simulink model "suspension_control_system"  (R2012b)
settings: Solver=ode3  SolverMode=SingleTasking  StartTime=0.0  StopTime=30  FixedStep=T  RelTol=1e-3
PreLoadFcn:
  | init_parameters;
undefined symbols (not defined in the file): K_lqr, opy_full, Suspension, sys_estimator
libraries: vehicle_dynamics_lib x7
settings Model: Creator=Marcus Sonntag  LastModifiedBy=vikafla
settings SolverCC: ZeroCrossAlgorithm=Adaptive
settings DataIOCC: SignalLoggingSaveFormat=ModelDataLogs  SaveOutput=off  SignalLogging=off  SaveTime=off
settings OptimizationCC: InlineParams=on  UseIntDivNetSlope=on  InlineInvariantSignals=on  EnhancedBackFolding=on  EfficientFloat2IntCast=on  SimCompilerOptimization=On
settings DebuggingCC: ArtificialAlgebraicLoopMsg=none  ParameterTunabilityLossMsg=none  FcnCallInpInsideContextMsg=UseLocalSettings  UniqueDataStoreMsg=error  StrictBusMsg=Warning
settings HardwareCC: ProdHWDeviceType=Generic->Unspecified (assume 32-bit Generic)  TargetIntDivRoundTo=Zero  TargetEndianess=LittleEndian  TargetHWDeviceType=Atmel->AVR
settings SFSimCC: SimParseCustomCode=off
settings RTWCC: SystemTargetFile=cn.tlc  TemplateMakefile=cn_msdll.tmf  PostCodeGenCommand=packNGo(buildInfo, {'packType' 'hierarchical'})  Description=Vector CANoe Real-Time Target DLL (Visual C/C++ Project Makefile)  ProcessScript=cn_make_rtw_hook  RTWCompilerOptimization=On
settings CodeAppCC: GenerateComments=off  MaxIdLength=128  SimulinkBlockComments=off
settings STFCustomTargetCC: CodeReplacementLibrary=ANSI_C  GeneratePreprocessorConditionals=Disable all  MatFileLogging=on  SystemTargetFile=cn.tlc
settings GRTTargetCC: ParMdlRefBuildCompliant=off  CompOptLevelCompliant=off  ConcurrentExecutionCompliant=off  CombineOutputUpdateFcns=off  GRTInterface=on  ExtModeMexFile=noextcomm  RTWCAPISignals=on  RTWCAPIParams=on

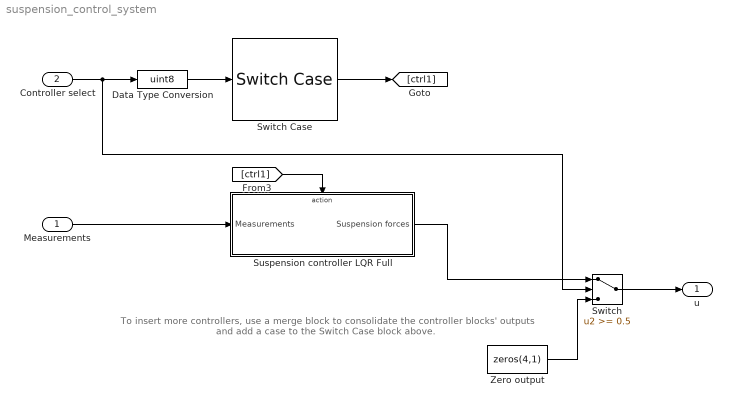
== system suspension_control_system ==
  note: To insert more controllers, use a merge block to consolidate
      | the controller blocks' outputs and add a case to the Switch Case
      | block above.
  Measurements : Inport  OutDataTypeStr=Bus: Bus_Measurements
  Controller select : Inport  Port=2
  Data Type Conversion : DataTypeConversion  OutDataTypeStr=uint8
  Suspension controller LQR Full : Subsystem
  Switch : Switch  Threshold=0.5
  Switch Case : SwitchCase  ShowDefaultCase=off
  Zero output : Constant  Value=zeros(4,1)
  u : Outport
  wires:
  Measurements/1 -> Suspension controller LQR Full/1(Measurements)
  Controller select/1 -> Data Type Conversion/1, Switch/2
  Switch Case/1 -> [ctrl1]
  [ctrl1] -> Suspension controller LQR Full/Action
  Data Type Conversion/1 -> Switch Case/1
  Suspension controller LQR Full/1(Suspension forces) -> Switch/1
  Switch/1 -> u/1
  Zero output/1 -> Switch/3

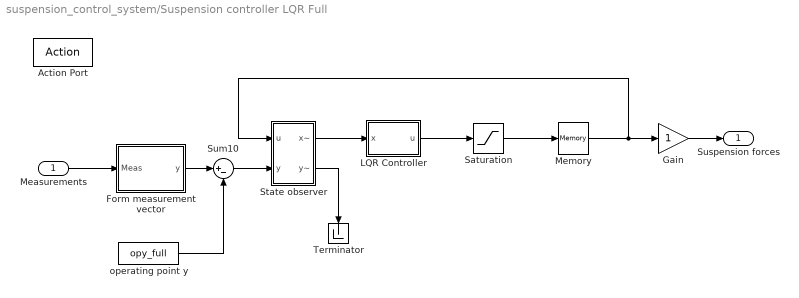
== system suspension_control_system/Suspension controller LQR Full ==
  Measurements : Inport
  Action Port : ActionPort  ActionType=case
  Form measurement vector : Subsystem
  Gain : Gain
  LQR Controller : Subsystem
  Memory : Memory
  Saturation : Saturate  UpperLimit=6e3  LowerLimit=-6e3
  State observer : Subsystem
  Sum10 : Sum  Inputs=|+-
  Terminator : Terminator
  operating point y : Constant  Value=opy_full
  Suspension forces : Outport  OutDataTypeStr=double  PortDimensions=4
  wires:
  LQR Controller/1(u) -> Saturation/1
  State observer/2(y~) -> Terminator/1
  Gain/1 -> Suspension forces/1
  State observer/1(x~) -> LQR Controller/1(x)
  Measurements/1 -> Form measurement vector/1(Meas)
  Form measurement vector/1(y) -> Sum10/1
  operating point y/1 -> Sum10/2
  Sum10/1 -> State observer/2(y)
  Saturation/1 -> Memory/1
  Memory/1 -> Gain/1, State observer/1(u)

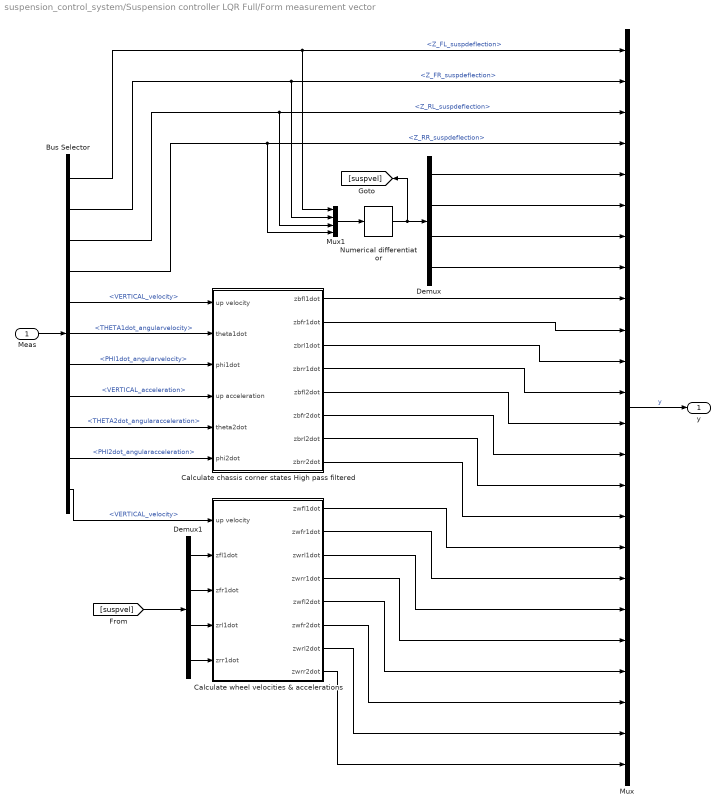
== system suspension_control_system/Suspension controller LQR Full/Form measurement vector ==
  Meas : Inport
  Bus Selector : BusSelector  OutputSignals=Z_FL_suspdeflection,Z_FR_suspdeflection,Z_RL_suspdeflection,Z_RR_suspdeflection,VERTICAL_velocity,THETA1dot_angularvelocity,PHI1dot_angularvelocity,VERTICAL_acceleration,THETA2dot_angularacceleration,PHI2dot_angularacceleration,VERTICAL_velocity
  Calculate chassis corner states High pass filtered : Subsystem
  Calculate wheel velocities & accelerations : Subsystem
  Demux : Demux
  Demux1 : Demux
  Mux : Mux  Inputs=24
  Mux1 : Mux
  Numerical differentiator : vehicle_dynamics_lib/Helper blocks/Numerical differentiator  SystemSampleTime=-1  Ts=0.01
  y : Outport
  wires:
  [suspvel] -> Demux1/1
  Demux1/4 -> Calculate wheel velocities & accelerations/5(zrr1dot)
  Demux1/3 -> Calculate wheel velocities & accelerations/4(zrl1dot)
  Demux1/2 -> Calculate wheel velocities & accelerations/3(zfr1dot)
  Demux1/1 -> Calculate wheel velocities & accelerations/2(zfl1dot)
  Demux/4 -> Mux/8
  Demux/3 -> Mux/7
  Demux/2 -> Mux/6
  Demux/1 -> Mux/5
  Numerical differentiator/1 -> [suspvel], Demux/1
  Mux1/1 -> Numerical differentiator/1
  Calculate wheel velocities & accelerations/8(zwrr2dot) -> Mux/24
  Calculate wheel velocities & accelerations/7(zwrl2dot) -> Mux/23
  Calculate wheel velocities & accelerations/6(zwfr2dot) -> Mux/22
  Calculate wheel velocities & accelerations/5(zwfl2dot) -> Mux/21
  Calculate wheel velocities & accelerations/4(zwrr1dot) -> Mux/20
  Calculate wheel velocities & accelerations/3(zwrl1dot) -> Mux/19
  Calculate wheel velocities & accelerations/2(zwfr1dot) -> Mux/18
  Calculate wheel velocities & accelerations/1(zwfl1dot) -> Mux/17
  Bus Selector/11 -> Calculate wheel velocities & accelerations/1(up velocity)  "<VERTICAL_velocity>"
  Calculate chassis corner states High pass filtered/8(zbrr2dot) -> Mux/16
  Calculate chassis corner states High pass filtered/7(zbrl2dot) -> Mux/15
  Calculate chassis corner states High pass filtered/6(zbfr2dot) -> Mux/14
  Calculate chassis corner states High pass filtered/5(zbfl2dot) -> Mux/13
  Calculate chassis corner states High pass filtered/4(zbrr1dot) -> Mux/12
  Calculate chassis corner states High pass filtered/3(zbrl1dot) -> Mux/11
  Calculate chassis corner states High pass filtered/2(zbfr1dot) -> Mux/10
  Calculate chassis corner states High pass filtered/1(zbfl1dot) -> Mux/9
  Bus Selector/10 -> Calculate chassis corner states High pass filtered/6(phi2dot)  "<PHI2dot_angularacceleration>"
  Bus Selector/7 -> Calculate chassis corner states High pass filtered/3(phi1dot)  "<PHI1dot_angularvelocity>"
  Bus Selector/4 -> Mux1/4, Mux/4  "<Z_RR_suspdeflection>"
  Bus Selector/3 -> Mux1/3, Mux/3  "<Z_RL_suspdeflection>"
  Bus Selector/2 -> Mux1/2, Mux/2  "<Z_FR_suspdeflection>"
  Bus Selector/1 -> Mux1/1, Mux/1  "<Z_FL_suspdeflection>"
  Bus Selector/5 -> Calculate chassis corner states High pass filtered/1(up velocity)  "<VERTICAL_velocity>"
  Bus Selector/6 -> Calculate chassis corner states High pass filtered/2(theta1dot)  "<THETA1dot_angularvelocity>"
  Bus Selector/9 -> Calculate chassis corner states High pass filtered/5(theta2dot)  "<THETA2dot_angularacceleration>"
  Bus Selector/8 -> Calculate chassis corner states High pass filtered/4(up acceleration)  "<VERTICAL_acceleration>"
  Meas/1 -> Bus Selector/1
  Mux/1 -> y/1  "y"

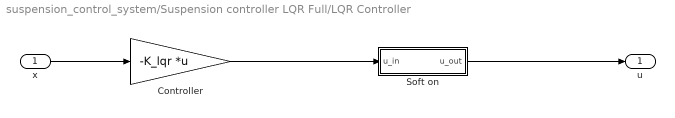
== system suspension_control_system/Suspension controller LQR Full/LQR Controller ==
  x : Inport  PortDimensions=14
  Controller : Gain  Gain=-K_lqr  Multiplication=Matrix(K*u)
  Soft on : Subsystem
  u : Outport
  wires:
  Soft on/1(u_out) -> u/1
  x/1 -> Controller/1
  Controller/1 -> Soft on/1(u_in)

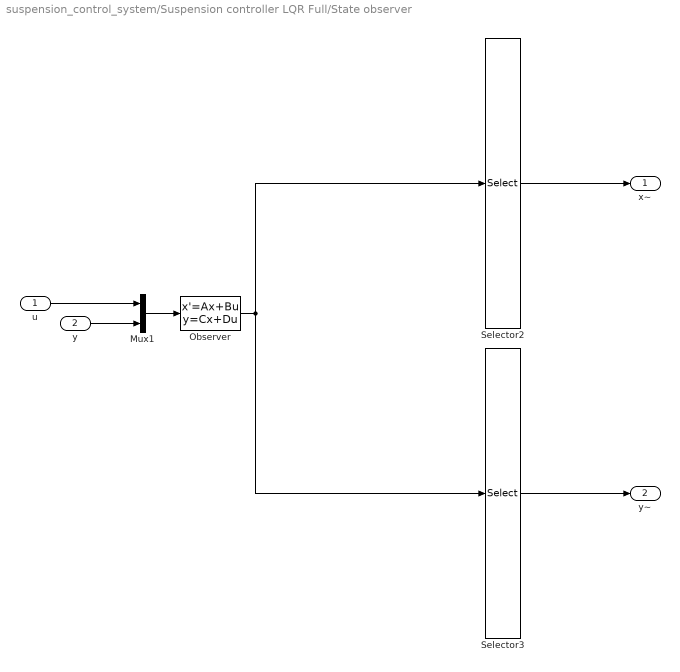
== system suspension_control_system/Suspension controller LQR Full/State observer ==
  u : Inport
  y : Inport  Port=2
  Mux1 : Mux  Inputs=2
  Observer : StateSpace  A=sys_estimator.A  B=sys_estimator.B  C=sys_estimator.C  D=sys_estimator.D  X0=zeros(14,1)
  Selector2 : Selector  InputPortWidth=size(sys_estimator.C,1)  IndexOptions=Index vector (dialog)  Indices=[(size(sys_estimator.C,1)-size(sys_estimator.A,1)+1):(size(sys_estimator.C,1))]  OutputSizes=1
  Selector3 : Selector  InputPortWidth=size(sys_estimator.C,1)  IndexOptions=Index vector (dialog)  Indices=[1:size(sys_estimator.C,1)-size(sys_estimator.A,1)]  OutputSizes=1
  x~ : Outport
  y~ : Outport  Port=2
  wires:
  Selector2/1 -> x~/1
  Selector3/1 -> y~/1
  Observer/1 -> Selector2/1, Selector3/1
  y/1 -> Mux1/2
  u/1 -> Mux1/1
  Mux1/1 -> Observer/1

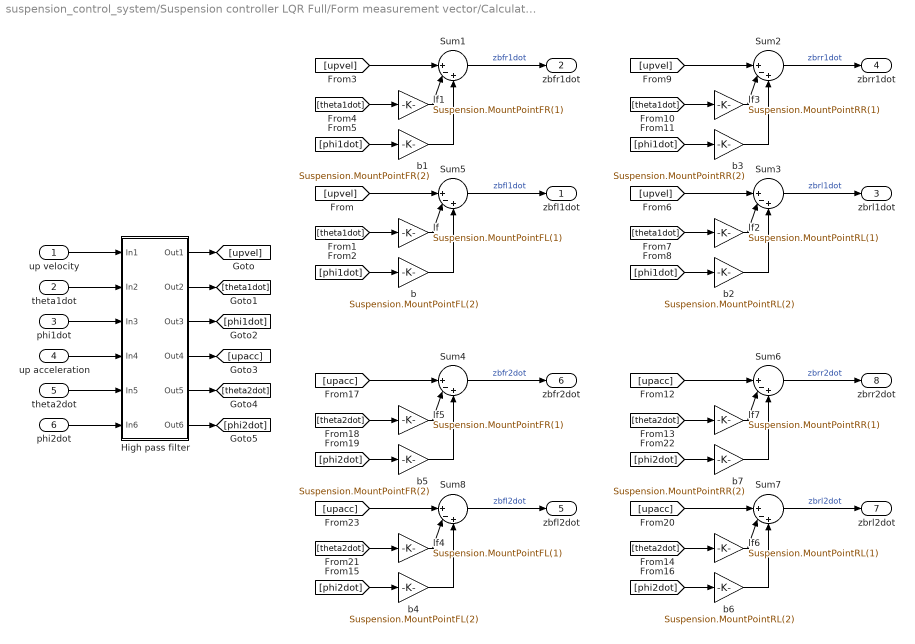
== system suspension_control_system/Suspension controller LQR Full/Form measurement vector/Calculate chassis corner states High pass filtered ==
  up velocity : Inport
  theta1dot : Inport  Port=2
  phi1dot : Inport  Port=3
  up acceleration : Inport  Port=4
  theta2dot : Inport  Port=5
  phi2dot : Inport  Port=6
  High pass filter : Subsystem
  Sum{1..8} (8 alike) : Sum  Inputs=||+-+
  b : Gain  Gain=Suspension.MountPointFL(2)
  b1 : Gain  Gain=Suspension.MountPointFR(2)
  b2 : Gain  Gain=Suspension.MountPointRL(2)
  b3 : Gain  Gain=Suspension.MountPointRR(2)
  b4 : Gain  Gain=Suspension.MountPointFL(2)
  b5 : Gain  Gain=Suspension.MountPointFR(2)
  b6 : Gain  Gain=Suspension.MountPointRL(2)
  b7 : Gain  Gain=Suspension.MountPointRR(2)
  lf : Gain  Gain=Suspension.MountPointFL(1)
  lf1 : Gain  Gain=Suspension.MountPointFR(1)
  lf2 : Gain  Gain=Suspension.MountPointRL(1)
  lf3 : Gain  Gain=Suspension.MountPointRR(1)
  lf4 : Gain  Gain=Suspension.MountPointFL(1)
  lf5 : Gain  Gain=Suspension.MountPointFR(1)
  lf6 : Gain  Gain=Suspension.MountPointRL(1)
  lf7 : Gain  Gain=Suspension.MountPointRR(1)
  zbfl1dot : Outport
  zbfr1dot : Outport  Port=2
  zbrl1dot : Outport  Port=3
  zbrr1dot : Outport  Port=4
  zbfl2dot : Outport  Port=5
  zbfr2dot : Outport  Port=6
  zbrl2dot : Outport  Port=7
  zbrr2dot : Outport  Port=8
  wires:
  [theta2dot] -> lf7/1
  [phi2dot] -> b7/1
  [upacc] -> Sum6/1
  b7/1 -> Sum6/3
  Sum6/1 -> zbrr2dot/1  "zbrr2dot"
  lf7/1 -> Sum6/2
  [theta2dot] -> lf6/1
  [phi2dot] -> b6/1
  [upacc] -> Sum7/1
  b6/1 -> Sum7/3
  Sum7/1 -> zbrl2dot/1  "zbrl2dot"
  lf6/1 -> Sum7/2
  [theta2dot] -> lf5/1
  [phi2dot] -> b5/1
  [upacc] -> Sum4/1
  b5/1 -> Sum4/3
  Sum4/1 -> zbfr2dot/1  "zbfr2dot"
  lf5/1 -> Sum4/2
  [theta2dot] -> lf4/1
  [phi2dot] -> b4/1
  [upacc] -> Sum8/1
  b4/1 -> Sum8/3
  Sum8/1 -> zbfl2dot/1  "zbfl2dot"
  lf4/1 -> Sum8/2
  High pass filter/6(Out6) -> [phi2dot]
  High pass filter/5(Out5) -> [theta2dot]
  High pass filter/4(Out4) -> [upacc]
  [theta1dot] -> lf3/1
  [phi1dot] -> b3/1
  [upvel] -> Sum2/1
  b3/1 -> Sum2/3
  Sum2/1 -> zbrr1dot/1  "zbrr1dot"
  lf3/1 -> Sum2/2
  [theta1dot] -> lf2/1
  [phi1dot] -> b2/1
  [upvel] -> Sum3/1
  b2/1 -> Sum3/3
  Sum3/1 -> zbrl1dot/1  "zbrl1dot"
  lf2/1 -> Sum3/2
  [theta1dot] -> lf1/1
  [phi1dot] -> b1/1
  [upvel] -> Sum1/1
  b1/1 -> Sum1/3
  Sum1/1 -> zbfr1dot/1  "zbfr1dot"
  lf1/1 -> Sum1/2
  [theta1dot] -> lf/1
  [phi1dot] -> b/1
  [upvel] -> Sum5/1
  High pass filter/3(Out3) -> [phi1dot]
  High pass filter/2(Out2) -> [theta1dot]
  High pass filter/1(Out1) -> [upvel]
  b/1 -> Sum5/3
  phi2dot/1 -> High pass filter/6(In6)
  theta2dot/1 -> High pass filter/5(In5)
  up acceleration/1 -> High pass filter/4(In4)
  phi1dot/1 -> High pass filter/3(In3)
  theta1dot/1 -> High pass filter/2(In2)
  up velocity/1 -> High pass filter/1(In1)
  Sum5/1 -> zbfl1dot/1  "zbfl1dot"
  lf/1 -> Sum5/2

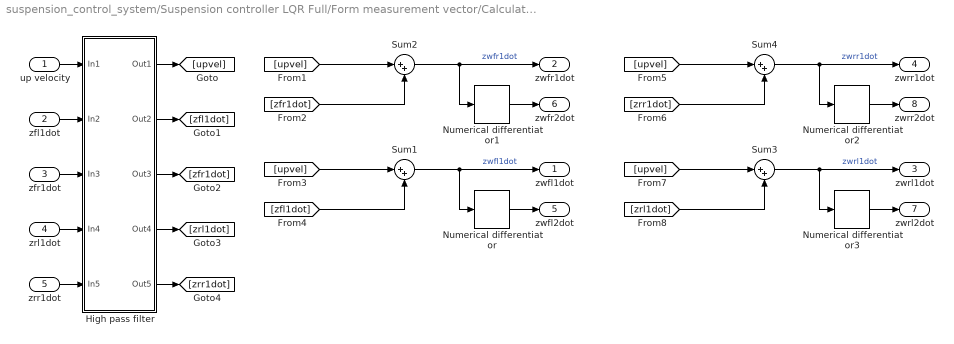
== system suspension_control_system/Suspension controller LQR Full/Form measurement vector/Calculate wheel velocities & accelerations ==
  up velocity : Inport
  zfl1dot : Inport  Port=2
  zfr1dot : Inport  Port=3
  zrl1dot : Inport  Port=4
  zrr1dot : Inport  Port=5
  High pass filter : Subsystem
  Numerical differentiator{,1..3} (4 alike) : vehicle_dynamics_lib/Helper blocks/Numerical differentiator  SystemSampleTime=-1  Ts=0.01
  Sum{1..4} (4 alike) : Sum  Inputs=|++
  zwfl1dot : Outport
  zwfr1dot : Outport  Port=2
  zwrl1dot : Outport  Port=3
  zwrr1dot : Outport  Port=4
  zwfl2dot : Outport  Port=5
  zwfr2dot : Outport  Port=6
  zwrl2dot : Outport  Port=7
  zwrr2dot : Outport  Port=8
  wires:
  High pass filter/5(Out5) -> [zrr1dot]
  High pass filter/4(Out4) -> [zrl1dot]
  High pass filter/3(Out3) -> [zfr1dot]
  High pass filter/2(Out2) -> [zfl1dot]
  High pass filter/1(Out1) -> [upvel]
  Numerical differentiator2/1 -> zwrr2dot/1
  Numerical differentiator3/1 -> zwrl2dot/1
  Numerical differentiator1/1 -> zwfr2dot/1
  Numerical differentiator/1 -> zwfl2dot/1
  Sum4/1 -> Numerical differentiator2/1, zwrr1dot/1  "zwrr1dot"
  [upvel] -> Sum4/1
  [zrr1dot] -> Sum4/2
  Sum3/1 -> Numerical differentiator3/1, zwrl1dot/1  "zwrl1dot"
  [upvel] -> Sum3/1
  [zrl1dot] -> Sum3/2
  Sum2/1 -> Numerical differentiator1/1, zwfr1dot/1  "zwfr1dot"
  [upvel] -> Sum2/1
  [zfr1dot] -> Sum2/2
  zrr1dot/1 -> High pass filter/5(In5)
  zrl1dot/1 -> High pass filter/4(In4)
  zfr1dot/1 -> High pass filter/3(In3)
  zfl1dot/1 -> High pass filter/2(In2)
  up velocity/1 -> High pass filter/1(In1)
  Sum1/1 -> Numerical differentiator/1, zwfl1dot/1  "zwfl1dot"
  [upvel] -> Sum1/1
  [zfl1dot] -> Sum1/2

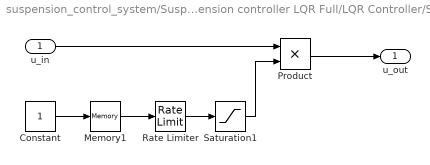
== system suspension_control_system/Suspension controller LQR Full/LQR Controller/Soft on ==
  u_in : Inport
  Constant : Constant  SampleTime=0
  Memory1 : Memory
  Product : Product  RndMeth=Zero
  Rate Limiter : RateLimiter  RisingSlewLimit=0.2  FallingSlewLimit=-inf  SampleTimeMode=inherited
  Saturation1 : Saturate  UpperLimit=1  LowerLimit=0
  u_out : Outport
  wires:
  Product/1 -> u_out/1
  Constant/1 -> Memory1/1
  u_in/1 -> Product/1
  Memory1/1 -> Rate Limiter/1
  Saturation1/1 -> Product/2
  Rate Limiter/1 -> Saturation1/1

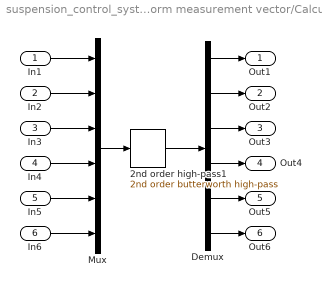
== system suspension_control_system/Suspension controller LQR Full/Form measurement vector/Calculate chassis corner states High pass filtered/High pass filter ==
  In1 : Inport
  In2 : Inport  Port=2
  In3 : Inport  Port=3
  In4 : Inport  Port=4
  In5 : Inport  Port=5
  In6 : Inport  Port=6
  2nd order high-pass1 : vehicle_dynamics_lib/Helper blocks/2nd order butterworth high-pass  SystemSampleTime=-1  wf=0.07  zeta=4.4
  Demux : Demux  Outputs=6
  Mux : Mux  Inputs=6
  Out1 : Outport
  Out2 : Outport  Port=2
  Out3 : Outport  Port=3
  Out4 : Outport  Port=4
  Out5 : Outport  Port=5
  Out6 : Outport  Port=6
  wires:
  2nd order high-pass1/1 -> Demux/1
  Demux/6 -> Out6/1
  Demux/5 -> Out5/1
  Demux/4 -> Out4/1
  Demux/3 -> Out3/1
  Demux/2 -> Out2/1
  Demux/1 -> Out1/1
  In6/1 -> Mux/6
  In5/1 -> Mux/5
  In4/1 -> Mux/4
  In3/1 -> Mux/3
  In2/1 -> Mux/2
  In1/1 -> Mux/1
  Mux/1 -> 2nd order high-pass1/1

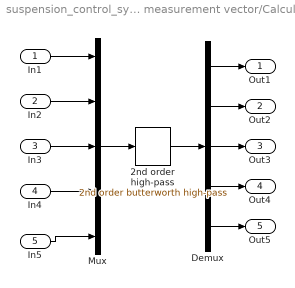
== system suspension_control_system/Suspension controller LQR Full/Form measurement vector/Calculate wheel velocities & accelerations/High pass filter ==
  In1 : Inport
  In2 : Inport  Port=2
  In3 : Inport  Port=3
  In4 : Inport  Port=4
  In5 : Inport  Port=5
  2nd order high-pass : vehicle_dynamics_lib/Helper blocks/2nd order butterworth high-pass  SystemSampleTime=-1  wf=0.07  zeta=4.4
  Demux : Demux  Outputs=5
  Mux : Mux  Inputs=5
  Out1 : Outport
  Out2 : Outport  Port=2
  Out3 : Outport  Port=3
  Out4 : Outport  Port=4
  Out5 : Outport  Port=5
  wires:
  2nd order high-pass/1 -> Demux/1
  Demux/5 -> Out5/1
  Demux/4 -> Out4/1
  Demux/3 -> Out3/1
  Demux/2 -> Out2/1
  Demux/1 -> Out1/1
  In5/1 -> Mux/5
  In4/1 -> Mux/4
  In3/1 -> Mux/3
  In2/1 -> Mux/2
  In1/1 -> Mux/1
  Mux/1 -> 2nd order high-pass/1
